simulink model "UART_read"  (R2024a)
settings: Solver=ode3  StartTime=0.0  StopTime=10  FixedStep=Ts  RelTol=1e-3
PostLoadFcn:
  | try
  | if isempty(which('ZHAWcbfcn'));
  | callback_fid07124=fopen('ZHAWcbfcn.m','w');
  | [~]=fprintf(callback_fid07124,'%s',get_param([bdroot,'/ Setup SLDRT'],'ClipboardFcn'));
  | [~]=fclose(callback_fid07124);
  | setpref('ZHAW_SLDRT_lib','cb_fcn',which('ZHAWcbfcn'))
  | clear callback_fid07124
  | end
  | catch
  | clear callback_fid07124
  | end
  | Ts=eval(get_param([bdroot,'/ Setup SLDRT'],'Ts'));
InitFcn:
  | Ts=eval(get_param([bdroot,'/ Setup SLDRT'],'Ts'));
undefined symbols (not defined in the file or in its folder): Serial_Port, Standard_Devices
libraries: sldrtlib x6, instrumentseriallib x2
(part 2 of 2)

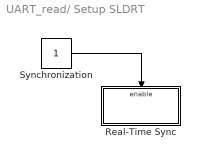
== system UART_read/ Setup SLDRT ==
  Real-Time Sync : Subsystem
  Synchronization : Constant
  wires:
  Synchronization/1 -> Real-Time Sync/Enable

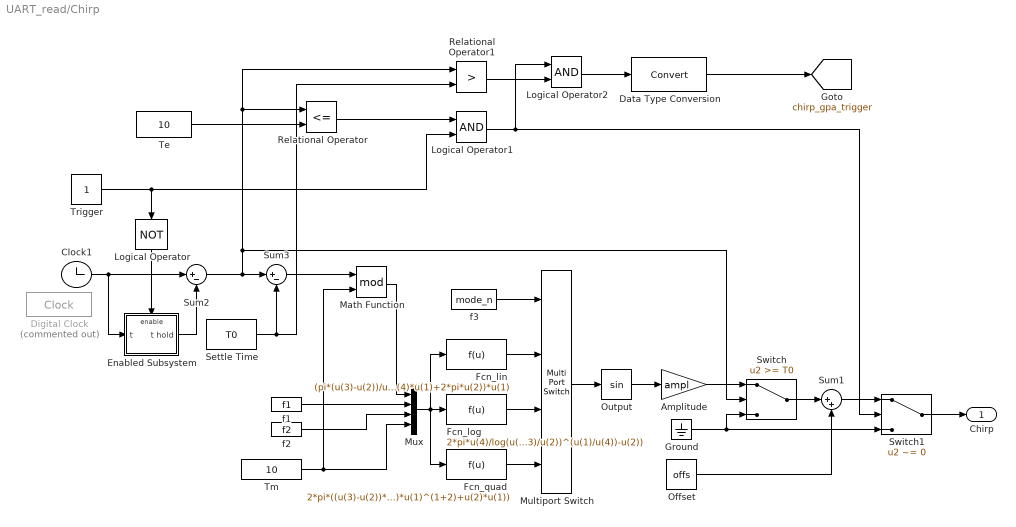
== system UART_read/Chirp ==
  Amplitude : Gain  Gain=ampl
  Clock1 : Clock
      settings: DisableCoverage=on
  Data Type Conversion : DataTypeConversion  SaturateOnIntegerOverflow=off  RndMeth=Floor
  Digital Clock : DigitalClock  Commented=on  SampleTime=Ts
  Enabled Subsystem : Subsystem  TreatAsAtomicUnit=on
  Fcn_lin : Fcn  Expr=(pi*(u(3)-u(2))/u(4)*u(1)+2*pi*u(2))*u(1)
  Fcn_log : Fcn  Expr=2*pi*u(4)/log(u(3)/u(2))*(u(2)*(u(3)/u(2))^(u(1)/u(4))-u(2))
  Fcn_quad : Fcn  Expr=2*pi*((u(3)-u(2))*u(4)^(-2)/(1+2)*u(1)^(1+2)+u(2)*u(1))
  Ground : Ground
  Logical Operator : Logic  Operator=NOT  AllPortsSameDT=off  OutDataTypeStr=boolean
  Logical Operator1 : Logic  AllPortsSameDT=off
  Logical Operator2 : Logic  AllPortsSameDT=off
  Math Function : Math  Operator=mod  SignedPower=on
  Multiport Switch : MultiPortSwitch  SaturateOnIntegerOverflow=off  InputSameDT=off
  Mux : Mux
  Offset : Constant  Value=offs
  Output : Trigonometry
  Relational Operator : RelationalOperator  Operator=<=  RndMeth=Simplest  InputSameDT=off
  Relational Operator1 : RelationalOperator  Operator=>  RndMeth=Simplest  InputSameDT=off
  Settle Time : Constant  Value=T0
  Sum1 : Sum  Inputs=|++
  Sum2 : Sum  Inputs=|+-
  Sum3 : Sum  Inputs=|+-
  Switch : Switch  Threshold=T0  SaturateOnIntegerOverflow=off  InputSameDT=off
  Switch1 : Switch  Criteria=u2 ~= 0  SaturateOnIntegerOverflow=off  InputSameDT=off
  Te : Constant  Value=10
  Tm : Constant  Value=10
  Trigger : Constant
  f1 : Constant  Value=f1
  f2 : Constant  Value=f2
  f3 : Constant  Value=mode_n
  Chirp : Outport  VectorParamsAs1DForOutWhenUnconnected=off
  tag scope: chirp_gpa_trigger=global
  wires:
  Te/1 -> Relational Operator/2
  Logical Operator/1 -> Enabled Subsystem/Enable
  Enabled Subsystem/1(t hold) -> Sum2/2
  Trigger/1 -> Logical Operator1/2, Logical Operator/1
  f3/1 -> Multiport Switch/1
  Fcn_lin/1 -> Multiport Switch/2
  Fcn_log/1 -> Multiport Switch/3
  Fcn_quad/1 -> Multiport Switch/4
  Multiport Switch/1 -> Output/1
  Math Function/1 -> Mux/1
  f2/1 -> Mux/3
  f1/1 -> Mux/2
  Mux/1 -> Fcn_log/1, Fcn_lin/1, Fcn_quad/1
  Clock1/1 -> Enabled Subsystem/1(t), Sum2/1
  Output/1 -> Amplitude/1
  Offset/1 -> Sum1/2
  Sum3/1 -> Math Function/1
  Tm/1 -> Mux/4, Math Function/2
  Switch/1 -> Sum1/1
  Amplitude/1 -> Switch/1
  Ground/1 -> Switch1/3, Switch/3
  Settle Time/1 -> Relational Operator1/2, Sum3/2
  Sum2/1 -> Switch/2, Relational Operator1/1, Relational Operator/1, Sum3/1
  Switch1/1 -> Chirp/1
  Sum1/1 -> Switch1/1
  Relational Operator/1 -> Logical Operator1/1
  Logical Operator1/1 -> Logical Operator2/1, Switch1/2
  Logical Operator2/1 -> Data Type Conversion/1
  Data Type Conversion/1 -> [chirp_gpa_trigger]
  Relational Operator1/1 -> Logical Operator2/2

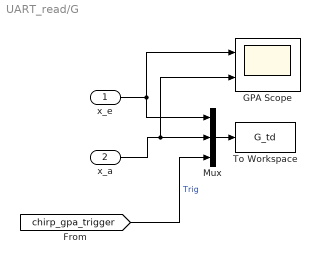
== system UART_read/G ==
  x_e : Inport
  x_a : Inport  Port=2
  GPA Scope : Scope  NumInputPorts=2
      settings: CopyFcn=try ZHAWcbfcn('copyScope'); end  NameChangeFcn=try ZHAWcbfcn('namechangeScope'); end
  Mux : Mux  Inputs=3
  To Workspace : ToWorkspace  VariableName=G_td  SaveFormat=Structure With Time  SampleTime=Ts
  wires:
  x_e/1 -> GPA Scope/1, Mux/1
  x_a/1 -> GPA Scope/2, Mux/2
  Mux/1 -> To Workspace/1
  [chirp_gpa_trigger] -> Mux/3  "Trig"

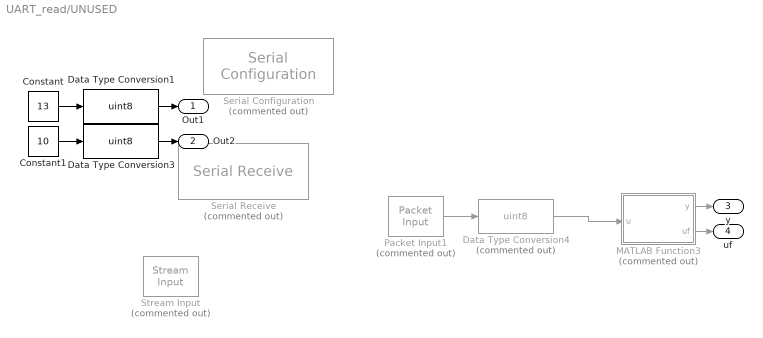
== system UART_read/UNUSED ==
  Constant : Constant  Value=13
  Constant1 : Constant  Value=10
  Data Type Conversion1 : DataTypeConversion  OutDataTypeStr=uint8  SaturateOnIntegerOverflow=off  RndMeth=Floor
  Data Type Conversion3 : DataTypeConversion  OutDataTypeStr=uint8  SaturateOnIntegerOverflow=off  RndMeth=Floor
  Data Type Conversion4 : DataTypeConversion  Commented=on  OutDataTypeStr=uint8  SaturateOnIntegerOverflow=off  RndMeth=Floor
  MATLAB Function3 : MATLAB Function  Commented=on  TreatAsAtomicUnit=on
  Packet Input1 : sldrtlib/Packet Input  Commented=on  SampleTime=Ts  MaxMissedTicks=10  ShowMissedTicks=off  YieldWhenWaiting=off  DrvName=Standard_Devices/Serial_Port  DrvAddress=27  DrvOptions=[460800 8 0 0 0 0 0 0]  PacketSize=6  DataTypes='6*uint8'  ShowReady=off  ShowError=off  PacketID=1  ByteOrder=1  ShowTimestamp=off
      settings: AttributesFormatString=Serial Port [27]
  Serial Configuration : instrumentseriallib/Serial Configuration  Priority=-200000  Commented=on  PortSel=COM27  Port=COM27  ComPort=COM27  BaudRate=460800  DataBits=8  Parity=none  StopBits=1  ByteOrder=little-endian  FlowControl=none  Timeout=10  SimulateUsing=Interpreted execution  BlockInModel=on  aMode=1
  Serial Receive : instrumentseriallib/Serial Receive  Priority=1  Commented=on  PortSel=COM27  Port=COM27  ComPort=COM27  DataType=uint8  SaveDataType=uint8  ToggleHeader=off  Header=[]  ToggleTerminator=off  Terminator=<none>  CustomTerminator=[]  InputFormat=Column major  ToggleDataSize=on  DataSize=[1 1]  EnableBlockingMode=off  ActionDataUnavailable=Output last received value  ActionWhenDataUnavailable=Output last received value  CustomValue=0  SampleTime=Ts  SimulateUsing=Interpreted execution  BlockInModel=on  aMode=1
  Stream Input : sldrtlib/Stream Input  Commented=on  SampleTime=Ts  MaxMissedTicks=Inf  ShowMissedTicks=off  YieldWhenWaiting=off  DrvName=Standard_Devices/Serial_Port  DrvAddress=27  DrvOptions=[460800 8 0 0 0 0 0 1]  DataTypes='uint8'  FormatString='%d'  Terminator='\n'  ShowReady=off  ShowError=on
      settings: AttributesFormatString=Serial Port [27]
  Out1 : Outport
  Out2 : Outport  Port=2
  y : Outport  Port=3
  uf : Outport  Port=4
  wires:
  Constant1/1 -> Data Type Conversion3/1
  Constant/1 -> Data Type Conversion1/1
  Data Type Conversion4/1 -> MATLAB Function3/1(u)
  MATLAB Function3/2(uf) -> uf/1
  MATLAB Function3/1(y) -> y/1
  Data Type Conversion3/1 -> Out2/1
  Packet Input1/1 -> Data Type Conversion4/1
  Data Type Conversion1/1 -> Out1/1

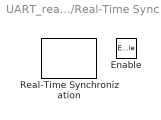
== system UART_read/ Setup SLDRT/Real-Time Sync ==
  Enable : EnablePort
  Real-Time Synchronization : sldrtlib/Real-Time Synchronization  SampleTime=Ts  MaxMissedTicks=inf  ShowMissedTicks=off  YieldWhenWaiting=off

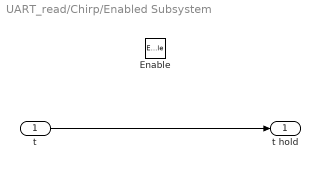
== system UART_read/Chirp/Enabled Subsystem ==
  t : Inport
  Enable : EnablePort
  t hold : Outport  VectorParamsAs1DForOutWhenUnconnected=off
  wires:
  t/1 -> t hold/1

== matlab function UART_read/UNUSED/MATLAB Function3 ==
  data: u input size=[6,1]; y output single size=[1,1]; uf output uint8 size=[4,1]
function [y,uf]   = fcn(u)
persistent old_u
if isempty(old_u)
    old_u = zeros(6,1,'uint8') ;
end
    n=find(u==10);
    nn=1:4;
    if ~isempty(n)
        switch n(1)
            case 1
                nn=(8:11)';
            case 2
                nn=(9:12)';
            case 3
                nn = [10 11 12 7]';
            case 4
                nn = [11 12 7 8]';
            case 5 
                nn = [12 7 8 9]';
            case 6
                nn = [7 8 9 10]';
            otherwise
                nn=(1:4)';
        end
    end
    %y=typecast(u(1:4),'single');
    %uf = u(1:4);
%else
    ug=([old_u;u]);
    y= typecast(ug([nn(1) nn(2) nn(3) nn(4)]),'single');
    uf= ug([nn(1) nn(2) nn(3) nn(4)]);
    old_u = u;
    %yf = typecast(y(:),'single');
%end
